simulink model "tr_trim_VTAOAS"  (R2025a)
settings: Solver=VariableStepAuto  StartTime=0.0  StopTime=10.0  RelTol=1e-3
values from neighbouring files (symbols this model uses):
  const = load_const    [vtol_trim_lin_analysis.m]
  q = X(8)    [fixedwing_6dof_dynamics.m]    (also in fixedwing_trim_dynamics.m; fw_linearization_dynamics.m; fw_trim_dynamics.m; tr_linearization_dynamics.m)
  r = X(9)    [fixedwing_6dof_dynamics.m]    (also in fixedwing_trim_dynamics.m; fw_linearization_dynamics.m; fw_trim_dynamics.m; tr_linearization_dynamics.m)
  uavParam = load_vtol_dynamics_7000lb    [vtol_trim_lin_analysis.m]
undefined symbols (not defined in the file or in its folder): contact, env, F, flap_trim, H_trim, Light, MIL, tiltIni, uavParams
libraries: matrix_library x8, robotcorelib x4, aerolibasang x2, aerolibwind2 x2, aerolibadyn x1, sharedutil x1, aerolibatmos2 x1, sharedtransform x1
(part 1 of 2)
settings Model: Creator=mhcho  LastModifiedBy=mhcho
settings DebuggingCC: InitInArrayFormatMsg=none

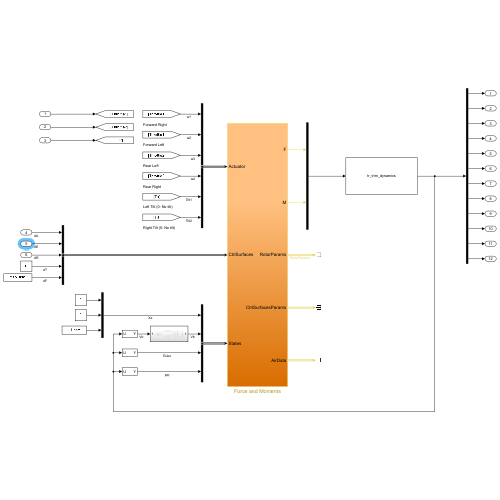
[thumbnail: Simulink's stored preview of the top-level diagram]
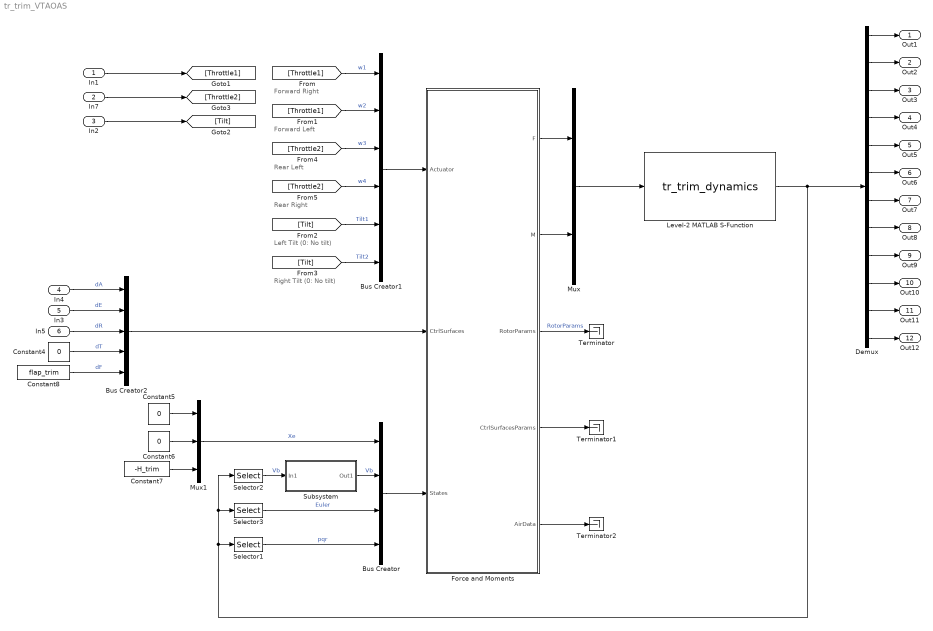
== system tr_trim_VTAOAS ==
  note: Forward Left
  note: Forward Right
  note: Rear Left
  note: Rear Right
  note: Left Tilt (0: No tilt)
  note: Right Tilt (0: No tilt)
  In1 : Inport
  In7 : Inport  Port=2
  In2 : Inport  Port=3
  In4 : Inport  Port=4
  In3 : Inport  Port=5
  In5 : Inport  Port=6
  Bus Creator : BusCreator  Inputs=4
  Bus Creator1 : BusCreator  Inputs=6  OutDataTypeStr=Bus: RotorCtrlBus
  Bus Creator2 : BusCreator  Inputs=5
  Constant4 : Constant  Value=0
  Constant5 : Constant  Value=0
  Constant6 : Constant  Value=0
  Constant7 : Constant  Value=-H_trim
  Constant8 : Constant  Value=flap_trim
  Demux : Demux  Outputs=12
  Force and Moments : Subsystem
  Level-2 MATLAB S-Function : M-S-Function  FunctionName=tr_trim_dynamics  Parameters=uavParams.geom.mass, uavParams.geom.Ixx, uavParams.geom.Iyy, uavParams.geom.Izz, uavParams.geom.Ixz, vt_trim, gamma_trim, const.g
  Mux : Mux  Inputs=2
  Mux1 : Mux  Inputs=3
  Selector1 : Selector  InputPortWidth=12  IndexOptions=Index vector (dialog)  Indices=[7 8 9]  OutputSizes=1
  Selector2 : Selector  InputPortWidth=12  IndexOptions=Index vector (dialog)  Indices=[1 2 3]  OutputSizes=1
  Selector3 : Selector  InputPortWidth=12  IndexOptions=Index vector (dialog)  Indices=[4 5 6]  OutputSizes=1
  Subsystem : Subsystem
  Terminator : Terminator
  Terminator1 : Terminator
  Terminator2 : Terminator
  Out1 : Outport
  Out2 : Outport  Port=2
  Out3 : Outport  Port=3
  Out4 : Outport  Port=4
  Out5 : Outport  Port=5
  Out6 : Outport  Port=6
  Out7 : Outport  Port=7
  Out8 : Outport  Port=8
  Out9 : Outport  Port=9
  Out10 : Outport  Port=10
  Out11 : Outport  Port=11
  Out12 : Outport  Port=12
  wires:
  [Tilt] -> Bus Creator1/6  "Tilt2"
  Bus Creator1/1 -> Force and Moments/1(Actuator)
  [Tilt] -> Bus Creator1/5  "Tilt1"
  Bus Creator2/1 -> Force and Moments/2(CtrlSurfaces)
  Force and Moments/1(F) -> Mux/1
  Force and Moments/2(M) -> Mux/2
  Mux/1 -> Level-2 MATLAB S-Function/1
  Bus Creator/1 -> Force and Moments/3(States)
  Demux/1 -> Out1/1
  Demux/2 -> Out2/1
  Mux1/1 -> Bus Creator/1  "Xe"
  Selector1/1 -> Bus Creator/4  "pqr"
  Selector3/1 -> Bus Creator/3  "Euler"
  Demux/3 -> Out3/1
  Demux/4 -> Out4/1
  Demux/5 -> Out5/1
  Demux/6 -> Out6/1
  Demux/7 -> Out7/1
  Demux/8 -> Out8/1
  Demux/9 -> Out9/1
  Demux/10 -> Out10/1
  Demux/11 -> Out11/1
  Demux/12 -> Out12/1
  Constant4/1 -> Bus Creator2/4  "dT"
  Constant5/1 -> Mux1/1
  Constant6/1 -> Mux1/2
  Constant7/1 -> Mux1/3
  [Throttle1] -> Bus Creator1/1  "w1"
  [Throttle1] -> Bus Creator1/2  "w2"
  Selector2/1 -> Subsystem/1(In1)  "Vb"
  Subsystem/1(Out1) -> Bus Creator/2  "Vb"
  Level-2 MATLAB S-Function/1 -> Selector1/1, Selector3/1, Selector2/1, Demux/1
  Force and Moments/3(RotorParams) -> Terminator/1  "RotorParams"
  Force and Moments/4(CtrlSurfacesParams) -> Terminator1/1
  In4/1 -> Bus Creator2/1  "dA"
  In3/1 -> Bus Creator2/2  "dE"
  In5/1 -> Bus Creator2/3  "dR"
  Force and Moments/5(AirData) -> Terminator2/1
  Constant8/1 -> Bus Creator2/5  "dF"
  [Throttle2] -> Bus Creator1/3  "w3"
  [Throttle2] -> Bus Creator1/4  "w4"
  In2/1 -> [Tilt]
  In7/1 -> [Throttle2]
  In1/1 -> [Throttle1]

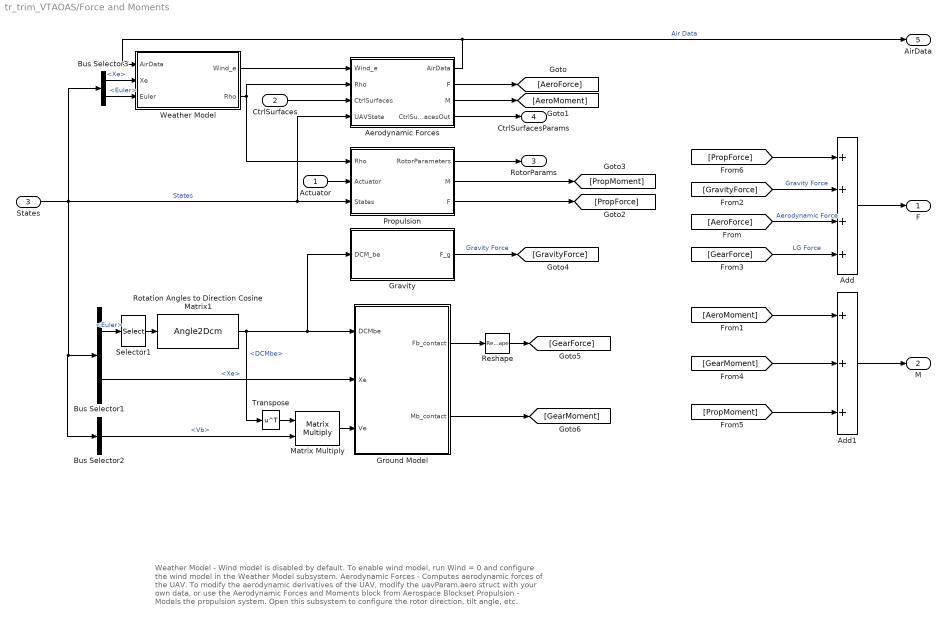
== system tr_trim_VTAOAS/Force and Moments ==
  note: Weather Model - Wind model is disabled by default. To enable wind model, run Wind = 0 and configure the wind model in the Weather Model subsystem.
      |
      | Aerodynamic Forces - Computes aerodynamic forces of the UAV. To modify the aerodynamic derivatives of the UAV, modify the uavParam.aero struct with your own data, or use the Aerodynamic Forces and Moments block from Aerospace Blockset
      |
      | Propulsion - Models the propulsion system. Open this subsystem to configure the rotor direction, tilt angle, etc.
  Actuator : Inport
  CtrlSurfaces : Inport  Port=2
  States : Inport  Port=3
  Add : Sum  Inputs=++++
  Add1 : Sum  Inputs=+++
  Aerodynamic Forces : Subsystem
  Bus Selector1 : BusSelector  OutputSignals=Euler,Xe
  Bus Selector2 : BusSelector  OutputSignals=Vb
  Bus Selector3 : BusSelector  OutputSignals=Xe,Euler
  Gravity : Subsystem
  Ground Model : Subsystem  VariantControl=Groundon==1
  Matrix Multiply : Product  Multiplication=Matrix(*)
  Propulsion : Subsystem
  Reshape : Reshape
  Rotation Angles to Direction Cosine Matrix1 : Angle2Dcm
      settings: AttributesFormatString=Rotation Order: %<rotationOrder>
  Selector1 : Selector  InputPortWidth=3  IndexOptions=Index vector (dialog)  Indices=[3 2 1]  OutputSizes=1
  Transpose : Math  Operator=transpose
  Weather Model : Subsystem  Variant=on  VariantControl=Weather Model
  F : Outport
  M : Outport  Port=2
  RotorParams : Outport  Port=3
  CtrlSurfacesParams : Outport  Port=4
  AirData : Outport  Port=5
  wires:
  [GravityForce] -> Add/2  "Gravity Force"
  Add/1 -> F/1
  CtrlSurfaces/1 -> Aerodynamic Forces/3(CtrlSurfaces)
  Add1/1 -> M/1
  [AeroForce] -> Add/3  "Aerodynamic Force"
  Aerodynamic Forces/2(F) -> [AeroForce]
  Actuator/1 -> Propulsion/2(Actuator)
  Propulsion/1(RotorParameters) -> RotorParams/1
  Aerodynamic Forces/1(AirData) -> Weather Model/1(AirData), AirData/1  "Air Data"
  Bus Selector3/1 -> Weather Model/2(Xe)  "<Xe>"
  Bus Selector3/2 -> Weather Model/3(Euler)  "<Euler>"
  Weather Model/1(Wind_e) -> Aerodynamic Forces/1(Wind_e)
  Weather Model/2(Rho) -> Propulsion/1(Rho), Aerodynamic Forces/2(Rho)
  Ground Model/1(Fb_contact) -> Reshape/1
  Aerodynamic Forces/3(M) -> [AeroMoment]
  Propulsion/3(F) -> [PropForce]
  Propulsion/2(M) -> [PropMoment]
  Gravity/1(F_g) -> [GravityForce]  "Gravity Force"
  Reshape/1 -> [GearForce]
  [GearForce] -> Add/4  "LG Force"
  Ground Model/2(Mb_contact) -> [GearMoment]
  [AeroMoment] -> Add1/1
  [GearMoment] -> Add1/2
  [PropMoment] -> Add1/3
  [PropForce] -> Add/1
  Aerodynamic Forces/4(CtrlSurfacesOut) -> CtrlSurfacesParams/1
  Bus Selector1/1 -> Selector1/1  "<Euler>"
  Bus Selector2/1 -> Matrix Multiply/2  "<Vb>"
  Rotation Angles to Direction Cosine Matrix1/1 -> Transpose/1, Gravity/1(DCM_be), Ground Model/1(DCMbe)  "<DCMbe>"
  Bus Selector1/2 -> Ground Model/2(Xe)  "<Xe>"
  Transpose/1 -> Matrix Multiply/1
  Selector1/1 -> Rotation Angles to Direction Cosine Matrix1/1
  States/1 -> Bus Selector2/1, Bus Selector1/1, Aerodynamic Forces/4(UAVState), Propulsion/3(States), Bus Selector3/1  "States"
  Matrix Multiply/1 -> Ground Model/3(Ve)

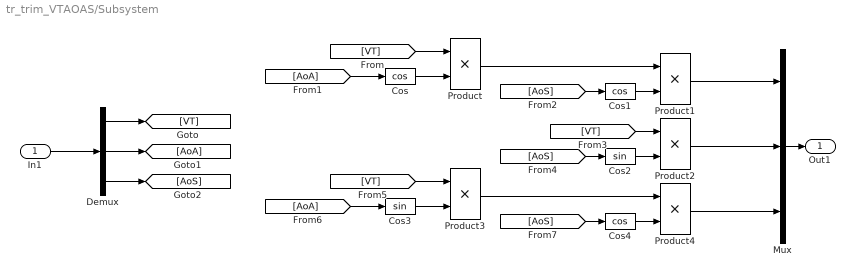
== system tr_trim_VTAOAS/Subsystem ==
  In1 : Inport
  Cos : Trigonometry  Operator=cos
  Cos1 : Trigonometry  Operator=cos
  Cos2 : Trigonometry
  Cos3 : Trigonometry
  Cos4 : Trigonometry  Operator=cos
  Demux : Demux  Outputs=3
  Mux : Mux  Inputs=3
  Product{,1..4} (5 alike) : Product
  Out1 : Outport
  wires:
  In1/1 -> Demux/1
  Demux/1 -> [VT]
  Demux/2 -> [AoA]
  Demux/3 -> [AoS]
  Mux/1 -> Out1/1
  [VT] -> Product/1
  Cos/1 -> Product/2
  [AoA] -> Cos/1
  Product/1 -> Product1/1
  Cos1/1 -> Product1/2
  [AoS] -> Cos1/1
  [VT] -> Product2/1
  [AoS] -> Cos2/1
  Cos2/1 -> Product2/2
  [AoA] -> Cos3/1
  [VT] -> Product3/1
  Cos3/1 -> Product3/2
  Product3/1 -> Product4/1
  [AoS] -> Cos4/1
  Cos4/1 -> Product4/2
  Product1/1 -> Mux/1
  Product2/1 -> Mux/2
  Product4/1 -> Mux/3

== system tr_trim_VTAOAS/Force and Moments/Aerodynamic Forces ==
  Wind_e : Inport
  Rho : Inport  Port=2
  CtrlSurfaces : Inport  Port=3
  UAVState : Inport  Port=4
  Bus Selector2 : BusSelector  OutputSignals=Euler,Vb,pqr
  Compute Air Data : Subsystem  TreatAsAtomicUnit=on  VariantControl=use_aerospace_blocks == 1
  Compute Body Frame Forces and Moments : Subsystem
  Matrix Multiply : Product  Multiplication=Matrix(*)
  Matrix Multiply1 : Product  Multiplication=Matrix(*)
  Rotation Angles to Direction Cosine Matrix1 : Angle2Dcm
      settings: AttributesFormatString=Rotation Order: %<rotationOrder>
  Selector1 : Selector  InputPortWidth=3  IndexOptions=Index vector (dialog)  Indices=[3 2 1]  OutputSizes=1
  Transpose : Math  Operator=transpose
  Vair : Sum  Inputs=+-  InputSameDT=on  SaturateOnIntegerOverflow=on  OutDataTypeStr=Inherit: Same as first input
  AirData : Outport  VectorParamsAs1DForOutWhenUnconnected=off
  F : Outport  Port=2
  M : Outport  Port=3
  CtrlSurfacesOut : Outport  Port=4
  wires:
  Compute Body Frame Forces and Moments/1(F_b) -> F/1
  CtrlSurfaces/1 -> Compute Body Frame Forces and Moments/2(CtrlSurfaces)
  Compute Air Data/1(AirData) -> Compute Body Frame Forces and Moments/1(AirData), AirData/1
  Compute Body Frame Forces and Moments/2(M_b) -> M/1
  Matrix Multiply/1 -> Compute Body Frame Forces and Moments/3(Vb), Compute Air Data/1(Vb)
  Rho/1 -> Compute Air Data/2(Rho)
  Vair/1 -> Matrix Multiply/2
  Wind_e/1 -> Vair/2
  Compute Body Frame Forces and Moments/3(CtrlSurfacesStates) -> CtrlSurfacesOut/1
  Bus Selector2/3 -> Compute Body Frame Forces and Moments/4(p,q,r)  "<pqr>"
  UAVState/1 -> Bus Selector2/1
  Matrix Multiply1/1 -> Vair/1
  Rotation Angles to Direction Cosine Matrix1/1 -> Matrix Multiply/1, Transpose/1  "<DCMbe>"
  Selector1/1 -> Rotation Angles to Direction Cosine Matrix1/1
  Transpose/1 -> Matrix Multiply1/1
  Bus Selector2/2 -> Matrix Multiply1/2  "<Vb>"
  Bus Selector2/1 -> Selector1/1  "<Euler>"

== system tr_trim_VTAOAS/Force and Moments/Gravity ==
  DCM_be : Inport
  Constant : Constant  Value=[0 0 const.g]'
  Gain : Gain  Gain=uavParams.geom.mass
  Matrix Multiply : Product  Multiplication=Matrix(*)
  F_g : Outport
  wires:
  Matrix Multiply/1 -> Gain/1
  Constant/1 -> Matrix Multiply/2
  DCM_be/1 -> Matrix Multiply/1
  Gain/1 -> F_g/1

== system tr_trim_VTAOAS/Force and Moments/Ground Model ==
  note: Body is assumed to be a rigid point mass on ground for contact force calculations.
      |
      | Normal force is modelled as a spring mass damper.
      |
      | Friction is modelled using Soft Coulomb model.
  note: #4, 25/05/20, MH, Not Fixed
      | Moment created by the landing gear is set to be
      | zero, which causes simulator divergence
      | Can be fixed by updating the tri-cycle landing
      | gear model
  DCMbe : Inport
  Xe : Inport  Port=2
  Ve : Inport  Port=3
  Constant : Constant  Value=[0 0 0]  SampleTime=-1
  Friction Force : Subsystem
  Matrix Multiply : Product  Multiplication=Matrix(*)
  Mux1 : Mux  Inputs=2
  Normal Force : Subsystem
  Selector : Selector  InputPortWidth=3  IndexOptions=Index vector (dialog)  Indices=[3]  OutputSizes=1
  Selector1 : Selector  InputPortWidth=3  IndexOptions=Index vector (dialog)  Indices=[3]  OutputSizes=1
  Selector2 : Selector  InputPortWidth=3  IndexOptions=Index vector (dialog)  Indices=[1,2]  OutputSizes=1
  Unary Minus1 : UnaryMinus
  Fb_contact : Outport
  Mb_contact : Outport  Port=2
  wires:
  Xe/1 -> Selector/1
  Ve/1 -> Selector2/1, Selector1/1
  Selector1/1 -> Normal Force/1(Vz)
  Selector/1 -> Normal Force/2(Z)
  DCMbe/1 -> Matrix Multiply/1
  Normal Force/1(Normal) -> Friction Force/2(Fn), Unary Minus1/1
  Unary Minus1/1 -> Mux1/2
  Selector2/1 -> Friction Force/1(V)
  Friction Force/1(Friction) -> Mux1/1
  Constant/1 -> Mb_contact/1
  Mux1/1 -> Matrix Multiply/2
  Matrix Multiply/1 -> Fb_contact/1

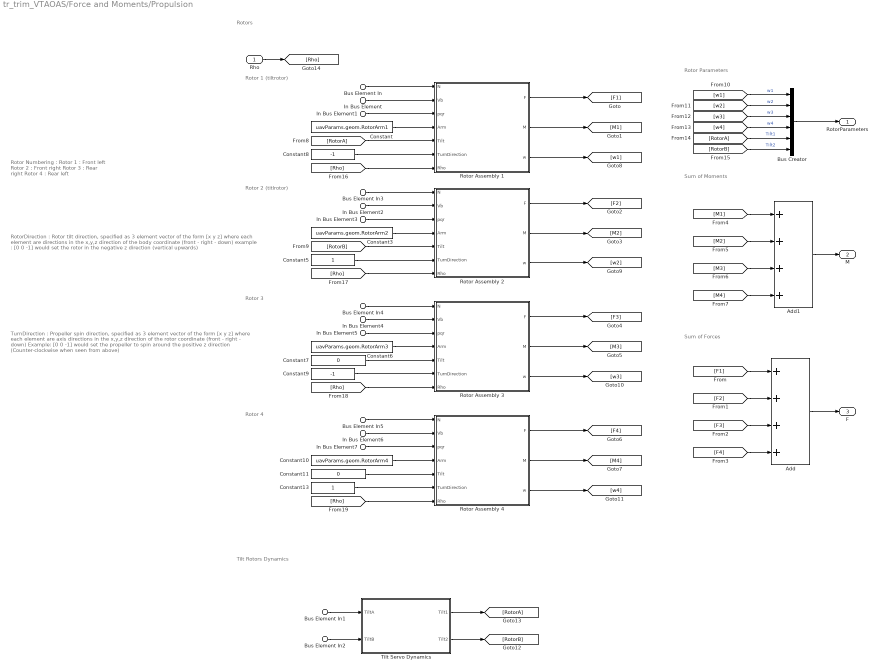
== system tr_trim_VTAOAS/Force and Moments/Propulsion ==
  note: TurnDirection : Propeller spin direction, specified as 3 element vector of the form [x y z] where each element are axis directions in the x,y,z direction of the rotor coordinate (front - right - down)
      |
      | Example: [0 0 -1] would set the propeller to spin around the positive z direction (Counter-clockwise when seen from above)
  note: RotorDirection : Rotor tilt direction, specified as 3 element vector of the form [x y z] where each element are directions in the x,y,z direction of the body coordinate (front - right - down)
      |
      | example : [0 0 -1] would set the rotor in the negative z direction (vertical upwards)
  note: Rotor Numbering :
      | Rotor 1 : Front left
      | Rotor 2 : Front right
      | Rotor 3 : Rear right
      | Rotor 4 : Rear left
  note: Tilt Rotors Dynamics
  note: Sum of Moments
  note: Rotor 1
      | (tiltrotor)
  note: Rotors
  note: Rotor 2
      | (titlrotor)
  note: Rotor 3
  note: Rotor 4
  note: Sum of Forces
  note: Rotor Parameters
  Rho : Inport
  Bus Element In : Inport  Port=2  PortName=Actuator  Element=w1
  Bus Element In1 : Inport  Port=2  PortName=Actuator  Element=Tilt1
  Bus Element In2 : Inport  Port=2  PortName=Actuator  Element=Tilt2
  Bus Element In3 : Inport  Port=2  PortName=Actuator  Element=w2
  Bus Element In5 : Inport  Port=2  PortName=Actuator  Element=w4
  Bus Element In4 : Inport  Port=2  PortName=Actuator  Element=w3
  In Bus Element{,2,4,6} (4 alike) : Inport  Port=3  PortName=States  Element=Vb
  In Bus Element{1,3,5,7} (4 alike) : Inport  Port=3  PortName=States  Element=pqr
  Add : Sum  Inputs=++++
  Add1 : Sum  Inputs=++++
  Bus Creator : BusCreator  Inputs=6  OutDataTypeStr=Bus: RotorCtrlBus
  Constant : Constant  Value=uavParams.geom.RotorArm1
  Constant10 : Constant  Value=uavParams.geom.RotorArm4
  Constant11 : Constant  Value=0
  Constant13 : Constant
  Constant3 : Constant  Value=uavParams.geom.RotorArm2
  Constant5 : Constant
  Constant6 : Constant  Value=uavParams.geom.RotorArm3
  Constant7 : Constant  Value=0
  Constant8 : Constant  Value=-1
  Constant9 : Constant  Value=-1
  Rotor Assembly 1 : Subsystem
  Rotor Assembly 2 : Subsystem
  Rotor Assembly 3 : Subsystem
  Rotor Assembly 4 : Subsystem
  Tilt Servo Dynamics : Subsystem
  RotorParameters : Outport
  M : Outport  Port=2
  F : Outport  Port=3
  wires:
  In Bus Element/1 -> Rotor Assembly 1/2(Vb)
  In Bus Element1/1 -> Rotor Assembly 1/3(pqr)
  Constant/1 -> Rotor Assembly 1/4(Arm)
  [RotorA] -> Rotor Assembly 1/5(Tilt)
  Add/1 -> F/1
  Constant8/1 -> Rotor Assembly 1/6(TurnDirection)
  Rotor Assembly 1/1(F) -> [F1]
  Rotor Assembly 1/2(M) -> [M1]
  Rotor Assembly 2/1(F) -> [F2]
  In Bus Element2/1 -> Rotor Assembly 2/2(Vb)
  Constant3/1 -> Rotor Assembly 2/4(Arm)
  Constant5/1 -> Rotor Assembly 2/6(TurnDirection)
  In Bus Element3/1 -> Rotor Assembly 2/3(pqr)
  Rotor Assembly 2/2(M) -> [M2]
  Rotor Assembly 3/1(F) -> [F3]
  In Bus Element4/1 -> Rotor Assembly 3/2(Vb)
  Constant6/1 -> Rotor Assembly 3/4(Arm)
  Constant9/1 -> Rotor Assembly 3/6(TurnDirection)
  Constant7/1 -> Rotor Assembly 3/5(Tilt)
  In Bus Element5/1 -> Rotor Assembly 3/3(pqr)
  Rotor Assembly 3/2(M) -> [M3]
  Rotor Assembly 4/1(F) -> [F4]
  In Bus Element6/1 -> Rotor Assembly 4/2(Vb)
  Constant10/1 -> Rotor Assembly 4/4(Arm)
  Constant13/1 -> Rotor Assembly 4/6(TurnDirection)
  Constant11/1 -> Rotor Assembly 4/5(Tilt)
  In Bus Element7/1 -> Rotor Assembly 4/3(pqr)
  Rotor Assembly 4/2(M) -> [M4]
  [F1] -> Add/1
  [F2] -> Add/2
  [F3] -> Add/3
  [F4] -> Add/4
  [M4] -> Add1/4
  Add1/1 -> M/1
  [M3] -> Add1/3
  [M2] -> Add1/2
  [M1] -> Add1/1
  [w1] -> Bus Creator/1  "w1"
  [w2] -> Bus Creator/2  "w2"
  [w3] -> Bus Creator/3  "w3"
  [w4] -> Bus Creator/4  "w4"
  Bus Creator/1 -> RotorParameters/1
  [RotorA] -> Bus Creator/5  "Tilt1"
  [RotorB] -> Bus Creator/6  "Tilt2"
  Bus Element In/1 -> Rotor Assembly 1/1(N)
  Bus Element In3/1 -> Rotor Assembly 2/1(N)
  Bus Element In4/1 -> Rotor Assembly 3/1(N)
  Bus Element In5/1 -> Rotor Assembly 4/1(N)
  Tilt Servo Dynamics/1(Tilt1) -> [RotorA]
  Tilt Servo Dynamics/2(Tilt2) -> [RotorB]
  Bus Element In1/1 -> Tilt Servo Dynamics/1(TiltA)
  Bus Element In2/1 -> Tilt Servo Dynamics/2(TiltB)
  Rotor Assembly 1/3(w) -> [w1]
  Rotor Assembly 2/3(w) -> [w2]
  Rho/1 -> [Rho]
  [Rho] -> Rotor Assembly 1/7(Rho)
  [RotorB] -> Rotor Assembly 2/5(Tilt)
  [Rho] -> Rotor Assembly 2/7(Rho)
  [Rho] -> Rotor Assembly 3/7(Rho)
  [Rho] -> Rotor Assembly 4/7(Rho)
  Rotor Assembly 3/3(w) -> [w3]
  Rotor Assembly 4/3(w) -> [w4]

== system tr_trim_VTAOAS/Force and Moments/Weather Model ==
  AirData : Inport
  Xe : Inport  Port=2
  Euler : Inport  Port=3
  Simple Model : Subsystem  VariantControl=Wind==0
  Weather Model : Subsystem  VariantControl=Wind==1
  Wind_e : Outport
  Rho : Outport  Port=2

== system tr_trim_VTAOAS/Force and Moments/Aerodynamic Forces/Compute Air Data ==
  Vb : Inport  PortDimensions=3
  Rho : Inport  Port=2
  Bus Creator : BusCreator  Inputs=4
  Dynamic Pressure : aerolibasang/Dynamic Pressure
  "Incidence, Sideslip, & Airspeed" : aerolibasang/Incidence, Sideslip, & Airspeed
  Saturation : Saturate  Commented=on  UpperLimit=max(uavParams.aero.beta_latdir)  LowerLimit=min(uavParams.aero.beta_latdir)
  Saturation1 : Saturate  Commented=on  UpperLimit=max(uavParams.aero.alpha_lon)  LowerLimit=min(uavParams.aero.alpha_lon)
  AirData : Outport  VectorParamsAs1DForOutWhenUnconnected=off
  wires:
  Bus Creator/1 -> AirData/1
  "Incidence, Sideslip, & Airspeed"/1 -> Bus Creator/1  "alpha"
  Rho/1 -> Dynamic Pressure/2
  "Incidence, Sideslip, & Airspeed"/3 -> Bus Creator/3  "airspeed"
  Dynamic Pressure/1 -> Bus Creator/4  "q"
  Vb/1 -> "Incidence, Sideslip, & Airspeed"/1, Dynamic Pressure/1
  "Incidence, Sideslip, & Airspeed"/2 -> Bus Creator/2  "beta"

== system tr_trim_VTAOAS/Force and Moments/Aerodynamic Forces/Compute Body Frame Forces and Moments ==
  note: Dynamic pressure
  note: #5, 25/06/09, MH, Working
      | Check which coordinate system OpenVSPAero
      | uses, probability body coordinate system
      | Set CP as the origin of aero analysis
      | Set CG obtained from OpenVSP
  note: Velocity in body axes
  note: Aerodynamic coefficients
  note: Dynamic pressure can be computed by using vehicle's velocity and air density
  AirData : Inport
  CtrlSurfaces : Inport  Port=2
  Vb : Inport  Port=3
  p,q,r : Inport  Port=4
  "Aerodynamic Forces and Moments " : aerolibadyn/Aerodynamic Forces and Moments   inputAxes=Wind  outputForceAxes=Body  outputMomentAxes=Body  S=uavParams.geom.b*uavParams.geom.c  b=uavParams.geom.b  cbar=uavParams.geom.c
  Constant1 : Constant  Value=[0 0 0]
  Constant2 : Constant  Value=[0 0 0]
  Wind frame F& M : Subsystem
  F_b : Outport  Unit=kg*m/s^2  VectorParamsAs1DForOutWhenUnconnected=off
  M_b : Outport  Port=2  Unit=kg*m/s  VectorParamsAs1DForOutWhenUnconnected=off
  CtrlSurfacesStates : Outport  Port=3  Unit=kg*m/s  VectorParamsAs1DForOutWhenUnconnected=off
  wires:
  p,q,r/1 -> Wind frame F& M/3(p,q,r)
  "Aerodynamic Forces and Moments "/2 -> M_b/1
  "Aerodynamic Forces and Moments "/1 -> F_b/1
  CtrlSurfaces/1 -> Wind frame F& M/2(CtrlSurfaces)
  AirData/1 -> Wind frame F& M/1(Airdata)
  Vb/1 -> "Aerodynamic Forces and Moments "/5
  Constant1/1 -> "Aerodynamic Forces and Moments "/3
  Constant2/1 -> "Aerodynamic Forces and Moments "/4
  Wind frame F& M/2(coef) -> "Aerodynamic Forces and Moments "/1  "FM_W"
  Wind frame F& M/3(q) -> "Aerodynamic Forces and Moments "/2
  Wind frame F& M/1(CtrlSurfacesStates) -> CtrlSurfacesStates/1

== system tr_trim_VTAOAS/Force and Moments/Ground Model/Friction Force ==
  V : Inport
  Fn : Inport  Port=2
  Product : Product
  Soft Coulomb Friction : Subsystem
  Unary Minus : UnaryMinus
  Friction : Outport
  wires:
  Unary Minus/1 -> Friction/1
  Fn/1 -> Product/2
  Soft Coulomb Friction/1(Out1) -> Product/1
  Product/1 -> Unary Minus/1
  V/1 -> Soft Coulomb Friction/1(V)

== system tr_trim_VTAOAS/Force and Moments/Ground Model/Normal Force ==
  Vz : Inport
  Z : Inport  Port=2
  Add : Sum
  Constant : Constant  Value=0  SampleTime=-1
  Damper : Gain  Gain=-sqrt(contact.spring*uavParams.geom.mass)
  Saturation : Saturate  UpperLimit=inf  LowerLimit=0  ZeroCross=off
  Spring Kp : Gain  Gain=-contact.spring
  Switch : Switch  Criteria=u2 > Threshold  SaturateOnIntegerOverflow=off  InputSameDT=off
  Unary Minus : UnaryMinus
  Unary Minus1 : UnaryMinus
  Normal : Outport
  wires:
  Add/1 -> Switch/3
  Constant/1 -> Switch/1
  Z/1 -> Unary Minus/1
  Switch/1 -> Saturation/1
  Damper/1 -> Add/2
  Spring Kp/1 -> Add/1
  Vz/1 -> Unary Minus1/1
  Saturation/1 -> Normal/1
  Unary Minus/1 -> Spring Kp/1, Switch/2
  Unary Minus1/1 -> Damper/1

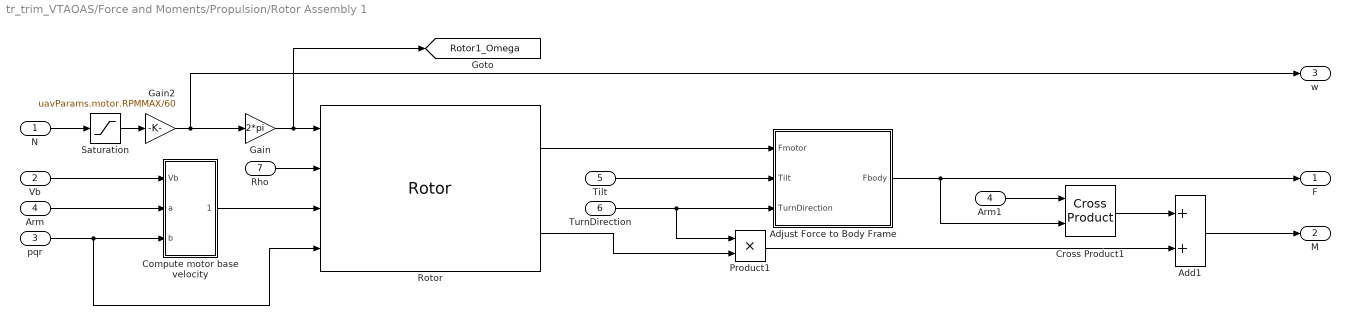
== system tr_trim_VTAOAS/Force and Moments/Propulsion/Rotor Assembly 1 ==
  N : Inport
  Vb : Inport  Port=2
  pqr : Inport  Port=3
  Arm : Inport  Port=4
  Tilt : Inport  Port=5
  TurnDirection : Inport  Port=6
  Rho : Inport  Port=7
  Add1 : Sum
  Adjust Force to Body Frame : Subsystem
  Arm1 : InportShadow  Port=4
  Compute motor base velocity : Subsystem
  Cross Product1 : matrix_library/Cross Product
  Gain : Gain  Gain=2*pi
  Gain2 : Gain  Gain=uavParams.motor.RPMMAX/60
  Product1 : Product
  Rotor : Rotor  modelMode=With flap effects  CT=uavParams.rotor.Ct  CQ=uavParams.rotor.Cq  Nb=uavParams.rotor.N  radius=uavParams.geom.PropDiameter/2  chord=uavParams.geom.PropChord  hingeOffset=uavParams.geom.PropOffHinge  clalpha=uavParams.geom.PropCLa  gamma=uavParams.geom.PropLock  thetaRoot=uavParams.geom.Propblroot  thetaTwist=uavParams.geom.Propbltwist
      settings: LibrarySourceBlock=aerolibrotor/Rotor
  Saturation : Saturate  UpperLimit=uavParams.motor.maxPWM  LowerLimit=uavParams.motor.minPWM
  F : Outport
  M : Outport  Port=2
  w : Outport  Port=3
  tag scope: Rotor1_Omega=global
  wires:
  TurnDirection/1 -> Adjust Force to Body Frame/3(TurnDirection), Product1/1
  Adjust Force to Body Frame/1(Fbody) -> F/1, Cross Product1/2
  Compute motor base velocity/1(Vmotor) -> Rotor/3
  Arm/1 -> Compute motor base velocity/2(a)
  Vb/1 -> Compute motor base velocity/1(Vb)
  Product1/1 -> Add1/2
  Cross Product1/1 -> Add1/1
  Arm1/1 -> Cross Product1/1
  Rho/1 -> Rotor/2
  Add1/1 -> M/1
  Rotor/2 -> Product1/2
  Gain/1 -> [Rotor1_Omega], Rotor/1
  pqr/1 -> Compute motor base velocity/3(b), Rotor/4
  Saturation/1 -> Gain2/1
  N/1 -> Saturation/1
  Tilt/1 -> Adjust Force to Body Frame/2(Tilt)
  Rotor/1 -> Adjust Force to Body Frame/1(Fmotor)
  Gain2/1 -> w/1, Gain/1

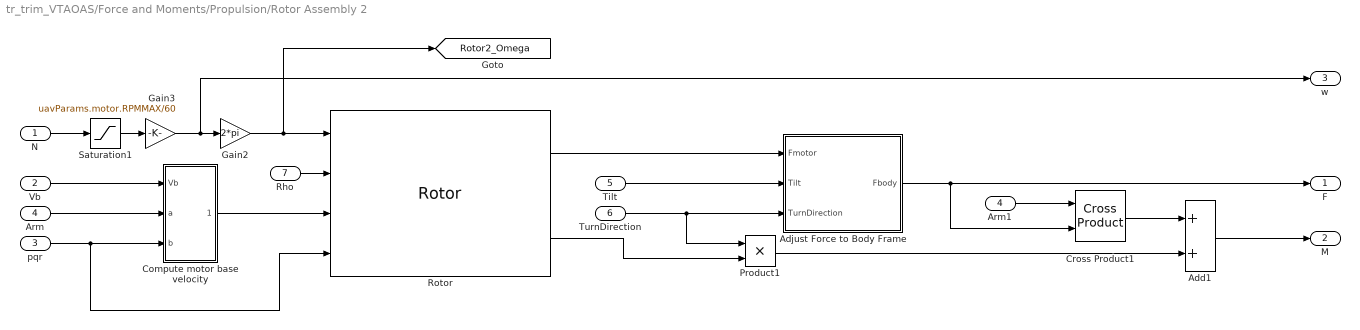
== system tr_trim_VTAOAS/Force and Moments/Propulsion/Rotor Assembly 2 ==
  N : Inport
  Vb : Inport  Port=2
  pqr : Inport  Port=3
  Arm : Inport  Port=4
  Tilt : Inport  Port=5
  TurnDirection : Inport  Port=6
  Rho : Inport  Port=7
  Add1 : Sum
  Adjust Force to Body Frame : Subsystem
  Arm1 : InportShadow  Port=4
  Compute motor base velocity : Subsystem
  Cross Product1 : matrix_library/Cross Product
  Gain2 : Gain  Gain=2*pi
  Gain3 : Gain  Gain=uavParams.motor.RPMMAX/60
  Product1 : Product
  Rotor : Rotor  modelMode=With flap effects  CT=uavParams.rotor.Ct  CQ=uavParams.rotor.Cq  Nb=uavParams.rotor.N  radius=uavParams.geom.PropDiameter/2  chord=uavParams.geom.PropChord  hingeOffset=uavParams.geom.PropOffHinge  clalpha=uavParams.geom.PropCLa  gamma=uavParams.geom.PropLock  thetaRoot=uavParams.geom.Propblroot  thetaTwist=uavParams.geom.Propbltwist
      settings: LibrarySourceBlock=aerolibrotor/Rotor
  Saturation1 : Saturate  UpperLimit=uavParams.motor.maxPWM  LowerLimit=uavParams.motor.minPWM
  F : Outport
  M : Outport  Port=2
  w : Outport  Port=3
  tag scope: Rotor2_Omega=global
  wires:
  TurnDirection/1 -> Adjust Force to Body Frame/3(TurnDirection), Product1/1
  Adjust Force to Body Frame/1(Fbody) -> F/1, Cross Product1/2
  Compute motor base velocity/1(Vmotor) -> Rotor/3
  Arm/1 -> Compute motor base velocity/2(a)
  Vb/1 -> Compute motor base velocity/1(Vb)
  Product1/1 -> Add1/2
  Cross Product1/1 -> Add1/1
  Arm1/1 -> Cross Product1/1
  Rho/1 -> Rotor/2
  Add1/1 -> M/1
  Rotor/2 -> Product1/2
  Gain2/1 -> [Rotor2_Omega], Rotor/1
  pqr/1 -> Compute motor base velocity/3(b), Rotor/4
  N/1 -> Saturation1/1
  Tilt/1 -> Adjust Force to Body Frame/2(Tilt)
  Rotor/1 -> Adjust Force to Body Frame/1(Fmotor)
  Gain3/1 -> Gain2/1, w/1
  Saturation1/1 -> Gain3/1

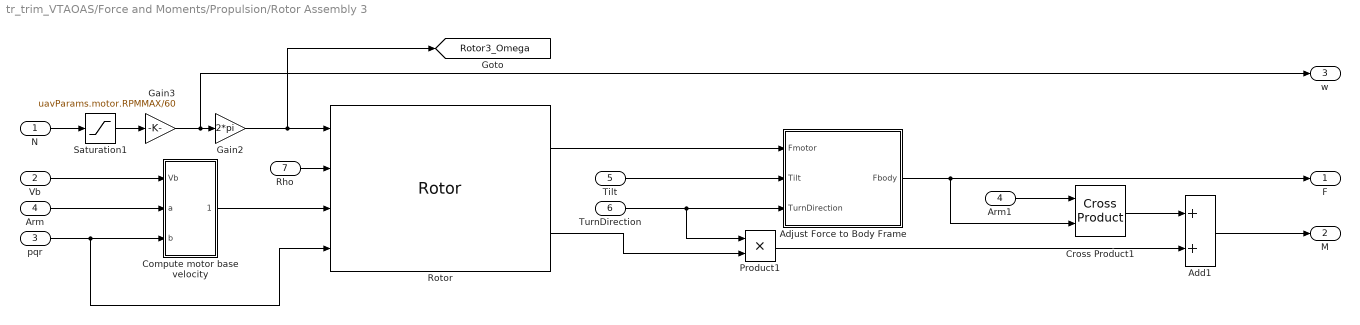
== system tr_trim_VTAOAS/Force and Moments/Propulsion/Rotor Assembly 3 ==
  N : Inport
  Vb : Inport  Port=2
  pqr : Inport  Port=3
  Arm : Inport  Port=4
  Tilt : Inport  Port=5
  TurnDirection : Inport  Port=6
  Rho : Inport  Port=7
  Add1 : Sum
  Adjust Force to Body Frame : Subsystem
  Arm1 : InportShadow  Port=4
  Compute motor base velocity : Subsystem
  Cross Product1 : matrix_library/Cross Product
  Gain2 : Gain  Gain=2*pi
  Gain3 : Gain  Gain=uavParams.motor.RPMMAX/60
  Product1 : Product
  Rotor : Rotor  modelMode=With flap effects  CT=uavParams.rotor.Ct  CQ=uavParams.rotor.Cq  Nb=uavParams.rotor.N  radius=uavParams.geom.PropDiameter/2  chord=uavParams.geom.PropChord  hingeOffset=uavParams.geom.PropOffHinge  clalpha=uavParams.geom.PropCLa  gamma=uavParams.geom.PropLock  thetaRoot=uavParams.geom.Propblroot  thetaTwist=uavParams.geom.Propbltwist
      settings: LibrarySourceBlock=aerolibrotor/Rotor
  Saturation1 : Saturate  UpperLimit=uavParams.motor.maxPWM  LowerLimit=uavParams.motor.minPWM
  F : Outport
  M : Outport  Port=2
  w : Outport  Port=3
  tag scope: Rotor3_Omega=global
  wires:
  TurnDirection/1 -> Adjust Force to Body Frame/3(TurnDirection), Product1/1
  Adjust Force to Body Frame/1(Fbody) -> F/1, Cross Product1/2
  Compute motor base velocity/1(Vmotor) -> Rotor/3
  Arm/1 -> Compute motor base velocity/2(a)
  Vb/1 -> Compute motor base velocity/1(Vb)
  Product1/1 -> Add1/2
  Cross Product1/1 -> Add1/1
  Arm1/1 -> Cross Product1/1
  Rho/1 -> Rotor/2
  Add1/1 -> M/1
  Rotor/2 -> Product1/2
  Gain2/1 -> [Rotor3_Omega], Rotor/1
  pqr/1 -> Compute motor base velocity/3(b), Rotor/4
  N/1 -> Saturation1/1
  Tilt/1 -> Adjust Force to Body Frame/2(Tilt)
  Rotor/1 -> Adjust Force to Body Frame/1(Fmotor)
  Gain3/1 -> Gain2/1, w/1
  Saturation1/1 -> Gain3/1

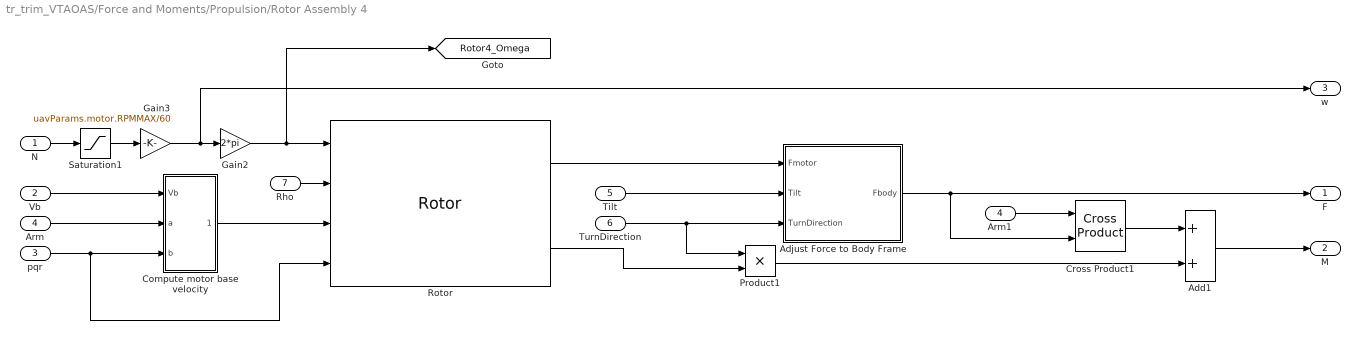
== system tr_trim_VTAOAS/Force and Moments/Propulsion/Rotor Assembly 4 ==
  N : Inport
  Vb : Inport  Port=2
  pqr : Inport  Port=3
  Arm : Inport  Port=4
  Tilt : Inport  Port=5
  TurnDirection : Inport  Port=6
  Rho : Inport  Port=7
  Add1 : Sum
  Adjust Force to Body Frame : Subsystem
  Arm1 : InportShadow  Port=4
  Compute motor base velocity : Subsystem
  Cross Product1 : matrix_library/Cross Product
  Gain2 : Gain  Gain=2*pi
  Gain3 : Gain  Gain=uavParams.motor.RPMMAX/60
  Product1 : Product
  Rotor : Rotor  modelMode=With flap effects  CT=uavParams.rotor.Ct  CQ=uavParams.rotor.Cq  Nb=uavParams.rotor.N  radius=uavParams.geom.PropDiameter/2  chord=uavParams.geom.PropChord  hingeOffset=uavParams.geom.PropOffHinge  clalpha=uavParams.geom.PropCLa  gamma=uavParams.geom.PropLock  thetaRoot=uavParams.geom.Propblroot  thetaTwist=uavParams.geom.Propbltwist
      settings: LibrarySourceBlock=aerolibrotor/Rotor
  Saturation1 : Saturate  UpperLimit=uavParams.motor.maxPWM  LowerLimit=uavParams.motor.minPWM
  F : Outport
  M : Outport  Port=2
  w : Outport  Port=3
  tag scope: Rotor4_Omega=global
  wires:
  TurnDirection/1 -> Adjust Force to Body Frame/3(TurnDirection), Product1/1
  Adjust Force to Body Frame/1(Fbody) -> F/1, Cross Product1/2
  Compute motor base velocity/1(Vmotor) -> Rotor/3
  Arm/1 -> Compute motor base velocity/2(a)
  Vb/1 -> Compute motor base velocity/1(Vb)
  Product1/1 -> Add1/2
  Cross Product1/1 -> Add1/1
  Arm1/1 -> Cross Product1/1
  Rho/1 -> Rotor/2
  Add1/1 -> M/1
  Rotor/2 -> Product1/2
  Gain2/1 -> [Rotor4_Omega], Rotor/1
  pqr/1 -> Compute motor base velocity/3(b), Rotor/4
  N/1 -> Saturation1/1
  Tilt/1 -> Adjust Force to Body Frame/2(Tilt)
  Rotor/1 -> Adjust Force to Body Frame/1(Fmotor)
  Gain3/1 -> Gain2/1, w/1
  Saturation1/1 -> Gain3/1

== system tr_trim_VTAOAS/Force and Moments/Propulsion/Tilt Servo Dynamics ==
  TiltA : Inport
  TiltB : Inport  Port=2
  Gain2 : Gain  Gain=pi/2
  Gain3 : Gain  Gain=pi/2
  IC : InitialCondition  Commented=through  Value=tiltIni
  IC1 : InitialCondition  Commented=through  Value=tiltIni
  Servo Dynamics : TransferFcn  Commented=through  Numerator=uavParams.tiltservo.tfnum  Denominator=uavParams.tiltservo.tfden
  Servo Dynamics1 : TransferFcn  Commented=through  Numerator=uavParams.tiltservo.tfnum  Denominator=uavParams.tiltservo.tfden
  Tilt1 : Outport
  Tilt2 : Outport  Port=2
  wires:
  Gain2/1 -> Servo Dynamics/1
  TiltB/1 -> Gain3/1
  Servo Dynamics/1 -> IC1/1
  Servo Dynamics1/1 -> IC/1
  IC/1 -> Tilt2/1  "Tilt2"
  IC1/1 -> Tilt1/1  "Tilt1"
  Gain3/1 -> Servo Dynamics1/1
  TiltA/1 -> Gain2/1

== system tr_trim_VTAOAS/Force and Moments/Weather Model/Simple Model ==
  note: #11, 25/07/04, MH, Fixed
      | Use International Standard Atmosphere model
      | to obtain the air density varying with altitude
  AirData : Inport
  Xe : Inport  Port=2
  Euler : Inport  Port=3
  Constant : Constant  Value=[ 0 0 0]
      settings: AttributesFormatString=%<Value>
  Constant1 : Constant  Commented=on  Value=const.rho0
  Gain : Gain  Gain=-1
  ISA Atmosphere Model : aerolibatmos2/ISA Atmosphere Model  useExtended=off  action=Warning  custom=off  viscosityOut=off  g=9.80665  gamma=1.4  R=287.0531  L=0.0065  h_trop=11000  h_strat=20000  rho0=1.225  P0=101325  T0=288.15  h0=0  S=110.4  Tref=273.15  muref=1.716e-5
  Selector : Selector  InputPortWidth=3  IndexOptions=Index vector (dialog)  Indices=[3]  OutputSizes=1
  Terminator{,1..4} (5 alike) : Terminator
  Wind_e : Outport  Unit=m/s  VectorParamsAs1DForOutWhenUnconnected=off
  " Rho" : Outport  Port=2  VectorParamsAs1DForOutWhenUnconnected=off
  wires:
  AirData/1 -> Terminator/1
  Constant/1 -> Wind_e/1
  Euler/1 -> Terminator1/1
  Xe/1 -> Selector/1
  Selector/1 -> Gain/1
  Gain/1 -> ISA Atmosphere Model/1
  ISA Atmosphere Model/1 -> Terminator2/1
  ISA Atmosphere Model/2 -> Terminator3/1
  ISA Atmosphere Model/3 -> Terminator4/1
  ISA Atmosphere Model/4 -> " Rho"/1

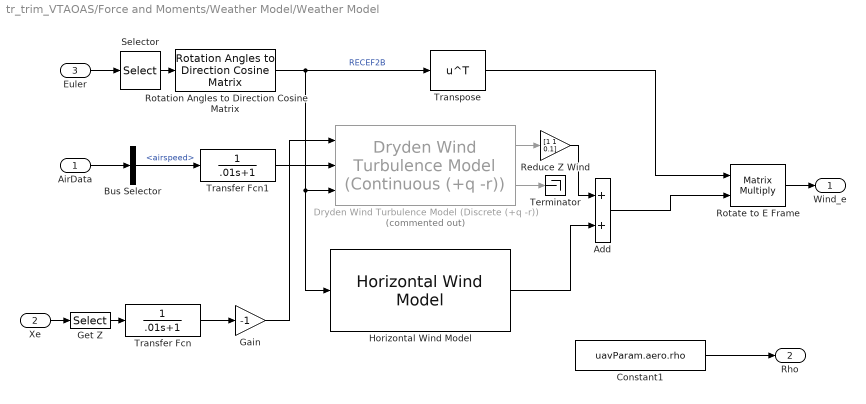
== system tr_trim_VTAOAS/Force and Moments/Weather Model/Weather Model ==
  AirData : Inport
  Xe : Inport  Port=2
  Euler : Inport  Port=3
  Add : Sum  Inputs=2
  Bus Selector : BusSelector  OutputSignals=airspeed
  Constant1 : Constant  Value=uavParam.aero.rho
  Dryden Wind Turbulence Model (Discrete (+q -r)) : aerolibwind2/Dryden Wind Turbulence Model  (Continuous (+q -r))  Commented=on  units=Metric (MKS)  spec=MIL-F-8785C  model=Discrete Dryden (+q -r)  W20=env.windBase/4  Wdeg=env.windDirTurb  TurbProb=10^-2 - Light  L_high=533.4  Wingspan=uavParam.geom.b  ts=0.005  Seed=[23341 23342 23343 23344]  T_on=on
  Gain : Gain  Gain=-1
      settings: AttributesFormatString=Z to Alt
  Get Z : Selector  InputPortWidth=3  IndexOptions=Index vector (dialog)  Indices=[3]  OutputSizes=[(-2)]
  Horizontal Wind Model : aerolibwind2/Horizontal Wind Model  units=Metric (MKS)  Vw_source=Internal  Vwind=8  W_source=Internal  Wdeg=env.windDirHor
  Reduce Z Wind : Gain  Gain=[1 1 0.1]
      settings: AttributesFormatString=%<Gain>
  Rotate to E Frame : Product  Multiplication=Matrix(*)
  Rotation Angles to Direction Cosine Matrix : sharedtransform/Rotation Angles to Direction Cosine Matrix  rotationOrder=ZYX  aMode=aMode
  Selector : Selector  InputPortWidth=3  IndexOptions=Index vector (dialog)  Indices=[3 2 1]  OutputSizes=1
  Terminator : Terminator
  Transfer Fcn : TransferFcn  Denominator=[.01 1]
  Transfer Fcn1 : TransferFcn  Denominator=[.01 1]
  Transpose : Math  Operator=transpose  SignedPower=on
  Wind_e : Outport  Unit=m/s  VectorParamsAs1DForOutWhenUnconnected=off
  Rho : Outport  Port=2  VectorParamsAs1DForOutWhenUnconnected=off
  wires:
  Bus Selector/1 -> Transfer Fcn1/1  "<airspeed>"
  AirData/1 -> Bus Selector/1
  Transfer Fcn/1 -> Gain/1
  Dryden Wind Turbulence Model (Discrete (+q -r))/2 -> Terminator/1
  Reduce Z Wind/1 -> Add/1
  Dryden Wind Turbulence Model (Discrete (+q -r))/1 -> Reduce Z Wind/1
  Rotate to E Frame/1 -> Wind_e/1
  Transpose/1 -> Rotate to E Frame/1
  Horizontal Wind Model/1 -> Add/2
  Transfer Fcn1/1 -> Dryden Wind Turbulence Model (Discrete (+q -r))/2
  Add/1 -> Rotate to E Frame/2
  Rotation Angles to Direction Cosine Matrix/1 -> Dryden Wind Turbulence Model (Discrete (+q -r))/3, Horizontal Wind Model/1, Transpose/1  "RECEF2B"
  Get Z/1 -> Transfer Fcn/1
  Xe/1 -> Get Z/1
  Gain/1 -> Dryden Wind Turbulence Model (Discrete (+q -r))/1
  Constant1/1 -> Rho/1
  Selector/1 -> Rotation Angles to Direction Cosine Matrix/1
  Euler/1 -> Selector/1

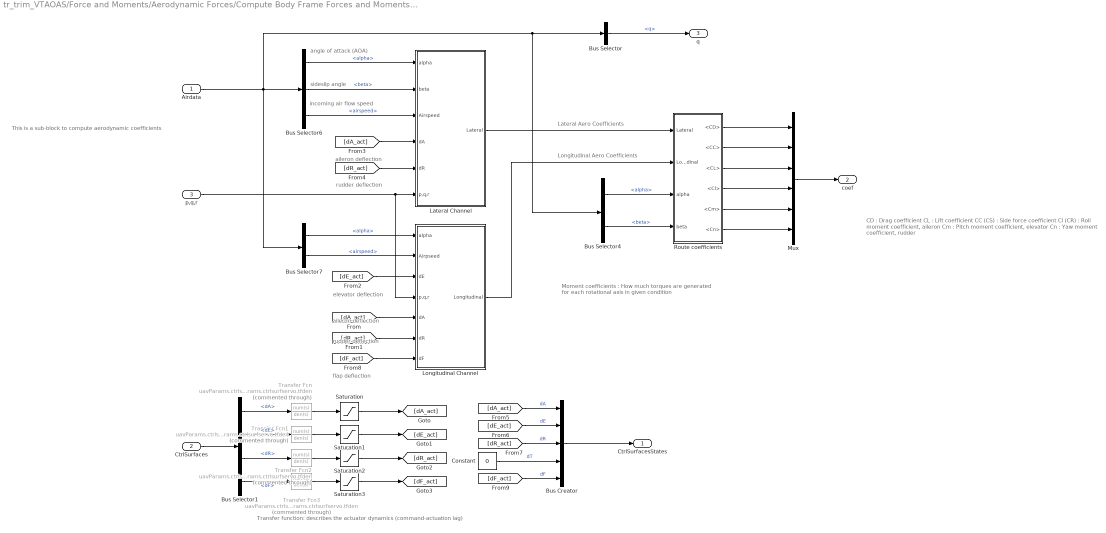
== system tr_trim_VTAOAS/Force and Moments/Aerodynamic Forces/Compute Body Frame Forces and Moments/Wind frame F& M ==
  note: CD : Drag coefficient
      | CL : Lift coefficient
      | CC (CS) : Side force coefficient
      | Cl (CR) : Roll moment coefficient, aileron
      | Cm : Pitch moment coefficient, elevator
      | Cn : Yaw moment coefficient, rudder
  note: Transfer function: describes the actuator dynamics (command-actuation lag)
  note: aileron deflection
  note: This is a sub-block to compute aerodynamic coefficients
  note: angle of attack (AOA)
  note: sideslip angle
  note: rudder deflection
  note: elevator deflection
  note: Lateral Aero Coefficients
  note: Longitudinal Aero Coefficients
  note: rudder deflection
  note: aileron deflection
  note: Moment coefficients : How much torques are generated for each rotational axis in given condition
  note: incoming air flow speed
  note: flap deflection
  Airdata : Inport
  CtrlSurfaces : Inport  Port=2
  p,q,r : Inport  Port=3
  Bus Creator : BusCreator  Inputs=5  OutDataTypeStr=Bus: FixedWingCtrlBus
  Bus Selector : BusSelector  OutputSignals=q
  Bus Selector1 : BusSelector  OutputSignals=dA,dE,dR,dF
  Bus Selector4 : BusSelector  OutputSignals=alpha,beta
  Bus Selector6 : BusSelector  OutputSignals=alpha,beta,airspeed
  Bus Selector7 : BusSelector  OutputSignals=alpha,airspeed
  Constant : Constant  Value=0
  Lateral Channel : Subsystem
  Longitudinal Channel : Subsystem
  Mux : Mux  Inputs=6
  Route coefficients : Subsystem
  Saturation : Saturate  UpperLimit=uavParams.maxAileron  LowerLimit=uavParams.minAileron
  Saturation1 : Saturate  UpperLimit=uavParams.maxElevator  LowerLimit=uavParams.minElevator
  Saturation2 : Saturate  UpperLimit=uavParams.maxRudder  LowerLimit=uavParams.minRudder
  Saturation3 : Saturate  UpperLimit=uavParams.maxFlap  LowerLimit=uavParams.minFlap
  Transfer Fcn{,1..3} (4 alike) : TransferFcn  Commented=through  Numerator=uavParams.ctrlsurfservo.tfnum  Denominator=uavParams.ctrlsurfservo.tfden
  CtrlSurfacesStates : Outport  VectorParamsAs1DForOutWhenUnconnected=off
  coef : Outport  Port=2  PortDimensions=6  VectorParamsAs1DForOutWhenUnconnected=off
  q : Outport  Port=3
  wires:
  Bus Selector7/2 -> Longitudinal Channel/2(Airpseed)  "<airspeed>"
  Bus Selector7/1 -> Longitudinal Channel/1(alpha)  "<alpha>"
  Bus Selector6/3 -> Lateral Channel/3(Airspeed)  "<airspeed>"
  Bus Selector6/2 -> Lateral Channel/2(beta)  "<beta>"
  Airdata/1 -> Bus Selector4/1, Bus Selector/1, Bus Selector7/1, Bus Selector6/1
  p,q,r/1 -> Longitudinal Channel/4(p,q,r), Lateral Channel/6(p,q,r)
  Mux/1 -> coef/1
  Longitudinal Channel/1(Longitudinal) -> Route coefficients/2(Longitudinal)
  Route coefficients/1(<CD>) -> Mux/1
  Route coefficients/2(<CC>) -> Mux/2
  Route coefficients/3(<CL>) -> Mux/3
  Route coefficients/4(<Cl>) -> Mux/4
  Route coefficients/5(<Cm>) -> Mux/5
  Route coefficients/6(<Cn>) -> Mux/6
  Bus Selector/1 -> q/1  "<q>"
  Lateral Channel/1(Lateral) -> Route coefficients/1(Lateral)
  Bus Selector4/1 -> Route coefficients/3(alpha)  "<alpha>"
  Bus Selector4/2 -> Route coefficients/4(beta)  "<beta>"
  Bus Selector6/1 -> Lateral Channel/1(alpha)  "<alpha>"
  Transfer Fcn/1 -> Saturation/1
  Transfer Fcn1/1 -> Saturation1/1
  Transfer Fcn2/1 -> Saturation2/1
  [dA_act] -> Longitudinal Channel/5(dA)
  [dR_act] -> Longitudinal Channel/6(dR)
  [dE_act] -> Longitudinal Channel/3(dE)
  [dA_act] -> Lateral Channel/4(dA)
  [dR_act] -> Lateral Channel/5(dR)
  CtrlSurfaces/1 -> Bus Selector1/1
  Bus Creator/1 -> CtrlSurfacesStates/1
  [dA_act] -> Bus Creator/1  "dA"
  [dE_act] -> Bus Creator/2  "dE"
  [dR_act] -> Bus Creator/3  "dR"
  Bus Selector1/1 -> Transfer Fcn/1  "<dA>"
  Bus Selector1/2 -> Transfer Fcn1/1  "<dE>"
  Bus Selector1/3 -> Transfer Fcn2/1  "<dR>"
  Saturation/1 -> [dA_act]
  Saturation2/1 -> [dR_act]
  Saturation1/1 -> [dE_act]
  Saturation3/1 -> [dF_act]
  Transfer Fcn3/1 -> Saturation3/1
  [dF_act] -> Longitudinal Channel/7(dF)
  Constant/1 -> Bus Creator/4  "dT"
  [dF_act] -> Bus Creator/5  "dF"
  Bus Selector1/4 -> Transfer Fcn3/1  "<dF>"

== system tr_trim_VTAOAS/Force and Moments/Ground Model/Friction Force/Soft Coulomb Friction ==
  note: Pennestrì, E., Rossi, V., Salvini, P. et al. Review and comparison of dry friction force models. Nonlinear Dyn 83, 1785–1801 (2016). https://doi.org/10.1007/s11071-015-2485-3
  V : Inport
  Tanh : Trigonometry  Operator=tanh
  friction coefficient : Gain  Gain=contact.rollingFriction*1.2
  vd : Gain  Gain=1/contact.vd
  Out1 : Outport
  wires:
  V/1 -> vd/1
  vd/1 -> Tanh/1
  Tanh/1 -> friction coefficient/1
  friction coefficient/1 -> Out1/1

== system tr_trim_VTAOAS/Force and Moments/Propulsion/Rotor Assembly 1/Adjust Force to Body Frame ==
  Fmotor : Inport
  Tilt : Inport  Port=2
  TurnDirection : Inport  Port=3
  Constant : Constant
  Constant1 : Constant
  Constant2 : Constant  Value=0
  Constant3 : Constant  Value=0
  Coordinate Transformation Conversion : robotcorelib/Coordinate Transformation Conversion  InputRepresentation=Euler Angles  InputEulerSequence=ZYX  ShowTrVecInputPort=on  OutputRepresentation=Rotation Matrix  OutputEulerSequence=ZYX  ShowTrVecOutputPort=on  SimulateUsing=Code generation
      settings: LibrarySourceBlock=uavutilslib/Coordinate Transformation Conversion
  Gain2 : Gain  Gain=-1
  Mux : Mux  Inputs=3
  Mux1 : Mux  Inputs=3
  Product : Product
  Product2 : Product  Multiplication=Matrix(*)
  Fbody : Outport
  wires:
  Constant1/1 -> Mux/3
  Constant/1 -> Mux/1
  Constant3/1 -> Mux1/3
  Constant2/1 -> Mux1/1
  Product2/1 -> Fbody/1
  Coordinate Transformation Conversion/1 -> Product2/1
  Mux/1 -> Product/2
  Product/1 -> Product2/2
  Gain2/1 -> Mux1/2
  TurnDirection/1 -> Mux/2
  Mux1/1 -> Coordinate Transformation Conversion/1
  Tilt/1 -> Gain2/1
  Fmotor/1 -> Product/1

== system tr_trim_VTAOAS/Force and Moments/Propulsion/Rotor Assembly 1/Compute motor base velocity ==
  Vb : Inport
  a : Inport  Port=2
  b : Inport  Port=3
  Add : Sum
  Cross Product : matrix_library/Cross Product
  Reshape : Reshape  OutputDimensionality=Column vector (2-D)
  Vmotor : Outport
  wires:
  b/1 -> Cross Product/2
  a/1 -> Cross Product/1
  Vb/1 -> Reshape/1
  Cross Product/1 -> Add/2
  Add/1 -> Vmotor/1
  Reshape/1 -> Add/1

== system tr_trim_VTAOAS/Force and Moments/Propulsion/Rotor Assembly 2/Adjust Force to Body Frame ==
  Fmotor : Inport
  Tilt : Inport  Port=2
  TurnDirection : Inport  Port=3
  Constant : Constant
  Constant1 : Constant
  Constant2 : Constant  Value=0
  Constant3 : Constant  Value=0
  Coordinate Transformation Conversion : robotcorelib/Coordinate Transformation Conversion  InputRepresentation=Euler Angles  InputEulerSequence=ZYX  ShowTrVecInputPort=on  OutputRepresentation=Rotation Matrix  OutputEulerSequence=ZYX  ShowTrVecOutputPort=on  SimulateUsing=Code generation
      settings: LibrarySourceBlock=uavutilslib/Coordinate Transformation Conversion
  Gain2 : Gain  Gain=-1
  Mux : Mux  Inputs=3
  Mux1 : Mux  Inputs=3
  Product : Product
  Product2 : Product  Multiplication=Matrix(*)
  Fbody : Outport
  wires:
  Constant1/1 -> Mux/3
  Constant/1 -> Mux/1
  Constant3/1 -> Mux1/3
  Constant2/1 -> Mux1/1
  Product2/1 -> Fbody/1
  Coordinate Transformation Conversion/1 -> Product2/1
  Mux/1 -> Product/2
  Product/1 -> Product2/2
  Gain2/1 -> Mux1/2
  TurnDirection/1 -> Mux/2
  Mux1/1 -> Coordinate Transformation Conversion/1
  Tilt/1 -> Gain2/1
  Fmotor/1 -> Product/1

== system tr_trim_VTAOAS/Force and Moments/Propulsion/Rotor Assembly 2/Compute motor base velocity ==
  Vb : Inport
  a : Inport  Port=2
  b : Inport  Port=3
  Add : Sum
  Cross Product : matrix_library/Cross Product
  Reshape : Reshape  OutputDimensionality=Column vector (2-D)
  Vmotor : Outport
  wires:
  b/1 -> Cross Product/2
  a/1 -> Cross Product/1
  Vb/1 -> Reshape/1
  Cross Product/1 -> Add/2
  Add/1 -> Vmotor/1
  Reshape/1 -> Add/1

== system tr_trim_VTAOAS/Force and Moments/Propulsion/Rotor Assembly 3/Adjust Force to Body Frame ==
  Fmotor : Inport
  Tilt : Inport  Port=2
  TurnDirection : Inport  Port=3
  Constant : Constant
  Constant1 : Constant
  Constant2 : Constant  Value=0
  Constant3 : Constant  Value=0
  Coordinate Transformation Conversion : robotcorelib/Coordinate Transformation Conversion  InputRepresentation=Euler Angles  InputEulerSequence=ZYX  ShowTrVecInputPort=on  OutputRepresentation=Rotation Matrix  OutputEulerSequence=ZYX  ShowTrVecOutputPort=on  SimulateUsing=Code generation
      settings: LibrarySourceBlock=uavutilslib/Coordinate Transformation Conversion
  Gain2 : Gain  Gain=-1
  Mux : Mux  Inputs=3
  Mux1 : Mux  Inputs=3
  Product : Product
  Product2 : Product  Multiplication=Matrix(*)
  Fbody : Outport
  wires:
  Constant1/1 -> Mux/3
  Constant/1 -> Mux/1
  Constant3/1 -> Mux1/3
  Constant2/1 -> Mux1/1
  Product2/1 -> Fbody/1
  Coordinate Transformation Conversion/1 -> Product2/1
  Mux/1 -> Product/2
  Product/1 -> Product2/2
  Gain2/1 -> Mux1/2
  TurnDirection/1 -> Mux/2
  Mux1/1 -> Coordinate Transformation Conversion/1
  Tilt/1 -> Gain2/1
  Fmotor/1 -> Product/1

== system tr_trim_VTAOAS/Force and Moments/Propulsion/Rotor Assembly 3/Compute motor base velocity ==
  Vb : Inport
  a : Inport  Port=2
  b : Inport  Port=3
  Add : Sum
  Cross Product : matrix_library/Cross Product
  Reshape : Reshape  OutputDimensionality=Column vector (2-D)
  Vmotor : Outport
  wires:
  b/1 -> Cross Product/2
  a/1 -> Cross Product/1
  Vb/1 -> Reshape/1
  Cross Product/1 -> Add/2
  Add/1 -> Vmotor/1
  Reshape/1 -> Add/1

== system tr_trim_VTAOAS/Force and Moments/Propulsion/Rotor Assembly 4/Adjust Force to Body Frame ==
  Fmotor : Inport
  Tilt : Inport  Port=2
  TurnDirection : Inport  Port=3
  Constant : Constant
  Constant1 : Constant
  Constant2 : Constant  Value=0
  Constant3 : Constant  Value=0
  Coordinate Transformation Conversion : robotcorelib/Coordinate Transformation Conversion  InputRepresentation=Euler Angles  InputEulerSequence=ZYX  ShowTrVecInputPort=on  OutputRepresentation=Rotation Matrix  OutputEulerSequence=ZYX  ShowTrVecOutputPort=on  SimulateUsing=Code generation
      settings: LibrarySourceBlock=uavutilslib/Coordinate Transformation Conversion
  Gain2 : Gain  Gain=-1
  Mux : Mux  Inputs=3
  Mux1 : Mux  Inputs=3
  Product : Product
  Product2 : Product  Multiplication=Matrix(*)
  Fbody : Outport
  wires:
  Constant1/1 -> Mux/3
  Constant/1 -> Mux/1
  Constant3/1 -> Mux1/3
  Constant2/1 -> Mux1/1
  Product2/1 -> Fbody/1
  Coordinate Transformation Conversion/1 -> Product2/1
  Mux/1 -> Product/2
  Product/1 -> Product2/2
  Gain2/1 -> Mux1/2
  TurnDirection/1 -> Mux/2
  Mux1/1 -> Coordinate Transformation Conversion/1
  Tilt/1 -> Gain2/1
  Fmotor/1 -> Product/1

== system tr_trim_VTAOAS/Force and Moments/Propulsion/Rotor Assembly 4/Compute motor base velocity ==
  Vb : Inport
  a : Inport  Port=2
  b : Inport  Port=3
  Add : Sum
  Cross Product : matrix_library/Cross Product
  Reshape : Reshape  OutputDimensionality=Column vector (2-D)
  Vmotor : Outport
  wires:
  b/1 -> Cross Product/2
  a/1 -> Cross Product/1
  Vb/1 -> Reshape/1
  Cross Product/1 -> Add/2
  Add/1 -> Vmotor/1
  Reshape/1 -> Add/1

== system tr_trim_VTAOAS/Force and Moments/Aerodynamic Forces/Compute Body Frame Forces and Moments/Wind frame F& M/Lateral Channel ==
  alpha : Inport
  beta : Inport  Port=2
  Airspeed : Inport  Port=3
  dA : Inport  Port=4
  dR : Inport  Port=5
  p,q,r : Inport  Port=6
  Bus Creator : BusCreator  Inputs=3
  CY : Subsystem
  Cl : Subsystem
  Cn : Subsystem
  Lateral : Outport  VectorParamsAs1DForOutWhenUnconnected=off
  wires:
  p,q,r/1 -> CY/4(p,q,r), Cl/5(p,q,r), Cn/5(p,q,r)
  Airspeed/1 -> CY/5(Airspeed), Cl/6(Airspeed), Cn/6(Airspeed)
  dR/1 -> CY/3(dR), Cl/4(dR), Cn/4(dR)
  dA/1 -> Cn/3(dA), Cl/3(dA)
  beta/1 -> CY/2(beta), Cn/2(beta), Cl/2(beta)
  Bus Creator/1 -> Lateral/1
  CY/1(CS) -> Bus Creator/1  "CS"
  alpha/1 -> Cl/1(alpha), Cn/1(alpha), CY/1(alpha)
  Cl/1(Cl) -> Bus Creator/2  "Cl"
  Cn/1(Cn) -> Bus Creator/3  "Cn"

== system tr_trim_VTAOAS/Force and Moments/Aerodynamic Forces/Compute Body Frame Forces and Moments/Wind frame F& M/Longitudinal Channel ==
  alpha : Inport
  Airpseed : Inport  Port=2
  dE : Inport  Port=3
  p,q,r : Inport  Port=4
  dA : Inport  Port=5
  dR : Inport  Port=6
  dF : Inport  Port=7
  Bus Creator : BusCreator  Inputs=3
  CD : Subsystem
  CL : Subsystem
  Cm : Subsystem
  Saturation : Saturate  UpperLimit=max(uavParams.aero.alpha_lon)  LowerLimit=min(uavParams.aero.alpha_lon)  ZeroCross=off
  Transfer Fcn : TransferFcn  Commented=on  Numerator=uavParams.aero.CLadot_tfnum  Denominator=uavParams.aero.CLadot_tfden
  Zero : Constant  Value=0  OutDataTypeStr=Inherit: Inherit via back propagation
  Longitudinal : Outport  VectorParamsAs1DForOutWhenUnconnected=off
  wires:
  Airpseed/1 -> Cm/4(Airspeed), CL/5(Airspeed)
  p,q,r/1 -> CL/4(p,q,r), Cm/3(p,q,r)
  Bus Creator/1 -> Longitudinal/1
  dE/1 -> CL/3(dE), Cm/2(dE), CD/4(dE)
  CD/1(CD) -> Bus Creator/1  "CD"
  alpha/1 -> Saturation/1
  dR/1 -> CD/3(dR)
  dA/1 -> CD/2(dA), CL/6(dA)
  Saturation/1 -> CD/1(alpha), Cm/1(alpha), CL/1(alpha), Transfer Fcn/1
  Cm/1(Cm) -> Bus Creator/3  "Cm"
  CL/1(CL) -> Bus Creator/2  "CL"
  dF/1 -> CD/5(dF), CL/7(dF), Cm/5(dF)
  Zero/1 -> CL/2(alpha_dot)

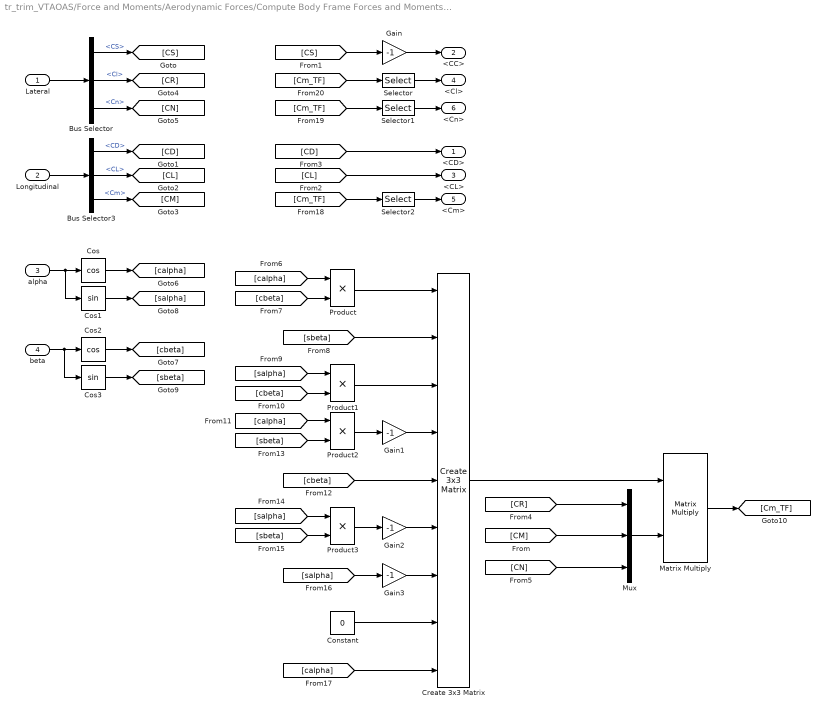
== system tr_trim_VTAOAS/Force and Moments/Aerodynamic Forces/Compute Body Frame Forces and Moments/Wind frame F& M/Route coefficients ==
  Lateral : Inport
  Longitudinal : Inport  Port=2
  alpha : Inport  Port=3
  beta : Inport  Port=4
  Bus Selector : BusSelector  OutputSignals=CS,Cl,Cn
  Bus Selector3 : BusSelector  OutputSignals=CD,CL,Cm
  Constant : Constant  Value=0
  Cos : Trigonometry  Operator=cos
  Cos1 : Trigonometry
  Cos2 : Trigonometry  Operator=cos
  Cos3 : Trigonometry
  Create 3x3 Matrix : sharedutil/Create 3x3 Matrix  aMode=aMode
      settings: LibrarySourceBlock=aerolibutil/Create 3x3 Matrix
  Gain{,1..3} (4 alike) : Gain  Gain=-1
  Matrix Multiply : Product  Multiplication=Matrix(*)
  Mux : Mux  Inputs=3
  Product{,1..3} (4 alike) : Product
  Selector : Selector  InputPortWidth=3  IndexOptions=Index vector (dialog)  Indices=[1]  OutputSizes=1
  Selector1 : Selector  InputPortWidth=3  IndexOptions=Index vector (dialog)  Indices=[3]  OutputSizes=1
  Selector2 : Selector  InputPortWidth=3  IndexOptions=Index vector (dialog)  Indices=[2]  OutputSizes=1
  <CD> : Outport
  <CC> : Outport  Port=2
  <CL> : Outport  Port=3
  <Cl> : Outport  Port=4
  <Cm> : Outport  Port=5
  <Cn> : Outport  Port=6
  wires:
  Lateral/1 -> Bus Selector/1
  Longitudinal/1 -> Bus Selector3/1
  Bus Selector/1 -> [CS]  "<CS>"
  Bus Selector3/1 -> [CD]  "<CD>"
  Bus Selector3/2 -> [CL]  "<CL>"
  [CL] -> <CL>/1
  [CD] -> <CD>/1
  Bus Selector3/3 -> [CM]  "<Cm>"
  Bus Selector/2 -> [CR]  "<Cl>"
  Bus Selector/3 -> [CN]  "<Cn>"
  Cos/1 -> [calpha]
  alpha/1 -> Cos1/1, Cos/1
  Cos1/1 -> [salpha]
  Cos2/1 -> [cbeta]
  Cos3/1 -> [sbeta]
  beta/1 -> Cos3/1, Cos2/1
  [calpha] -> Product/1
  [cbeta] -> Product/2
  Product/1 -> Create 3x3 Matrix/1
  [sbeta] -> Create 3x3 Matrix/2
  Product1/1 -> Create 3x3 Matrix/3
  [salpha] -> Product1/1
  [cbeta] -> Product1/2
  [calpha] -> Product2/1
  Product2/1 -> Gain1/1
  [sbeta] -> Product2/2
  Gain1/1 -> Create 3x3 Matrix/4
  [cbeta] -> Create 3x3 Matrix/5
  Product3/1 -> Gain2/1
  [salpha] -> Product3/1
  [sbeta] -> Product3/2
  Gain2/1 -> Create 3x3 Matrix/6
  Gain3/1 -> Create 3x3 Matrix/7
  [salpha] -> Gain3/1
  Constant/1 -> Create 3x3 Matrix/8
  [calpha] -> Create 3x3 Matrix/9
  Create 3x3 Matrix/1 -> Matrix Multiply/1
  Mux/1 -> Matrix Multiply/2
  [CM] -> Mux/2
  Matrix Multiply/1 -> [Cm_TF]
  [Cm_TF] -> Selector/1
  [Cm_TF] -> Selector1/1
  [Cm_TF] -> Selector2/1
  [CR] -> Mux/1
  [CN] -> Mux/3
  Gain/1 -> <CC>/1
  [CS] -> Gain/1
  Selector2/1 -> <Cm>/1
  Selector/1 -> <Cl>/1
  Selector1/1 -> <Cn>/1

== system tr_trim_VTAOAS/Force and Moments/Aerodynamic Forces/Compute Body Frame Forces and Moments/Wind frame F& M/Lateral Channel/CY ==
  alpha : Inport
  beta : Inport  Port=2
  dR : Inport  Port=3
  p,q,r : Inport  Port=4
  Airspeed : Inport  Port=5
  1-D Lookup Table : Lookup_n-D  BreakpointsForDimension1=uavParams.aero.beta_latdir  BreakpointsForDimension2=uavParams.aero.alpha_latdir  Table=uavParams.aero.CS  ExtrapMethod=Clip  UseLastTableValue=on  InternalRulePriority=Speed  RndMeth=Simplest
      settings: InputPortMap=u0,u1
  Abs : Abs  Commented=on  SaturateOnIntegerOverflow=off
  CYDr : Constant  Value=uavParams.aero.CYDr
      settings: AttributesFormatString=%<Value>
  CYb : Constant  Commented=on  Value=uavParam.aero.CYb
      settings: AttributesFormatString=%<Value>
  Product : Product  Commented=on  SaturateOnIntegerOverflow=on  OutDataTypeStr=Inherit: Same as first input
  Product1 : Product  SaturateOnIntegerOverflow=on  OutDataTypeStr=Inherit: Same as first input
  Product2 : Product  Commented=on
  Sign : Signum  Commented=on
  Sum2 : Sum  Inputs=++++  SaturateOnIntegerOverflow=on
  roll factors : Subsystem
  CS : Outport  VectorParamsAs1DForOutWhenUnconnected=off
  wires:
  dR/1 -> Product1/2
  CYDr/1 -> Product1/1
  CYb/1 -> Product/1
  Airspeed/1 -> roll factors/2(Airspeed)
  p,q,r/1 -> roll factors/1(p,q,r)
  Sum2/1 -> CS/1
  1-D Lookup Table/1 -> Sum2/1
  Sign/1 -> Product2/2
  Product1/1 -> Sum2/2
  roll factors/1(CSp) -> Sum2/3
  roll factors/2(CSr) -> Sum2/4
  beta/1 -> 1-D Lookup Table/1
  alpha/1 -> 1-D Lookup Table/2
